simulink model "LAB3"  (R2023a)
settings: Solver=VariableStepAuto  StartTime=0.0  StopTime=10.0  MaxStep=0.001  RelTol=1e-3
values from neighbouring files (symbols this model uses):
  K = 1.5    [LAB3.m]
  T = 0.5    [LAB3.m]
  Wn = 8    [LAB3.m]
  Zeta = 1    [LAB3.m]
settings Model: Creator=alaam  LastModifiedBy=alaam

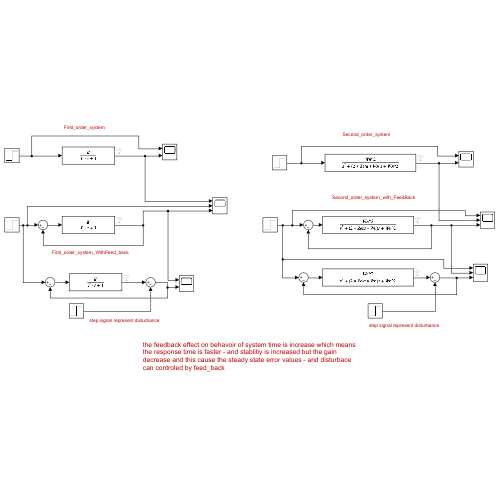
[thumbnail: Simulink's stored preview of the top-level diagram]
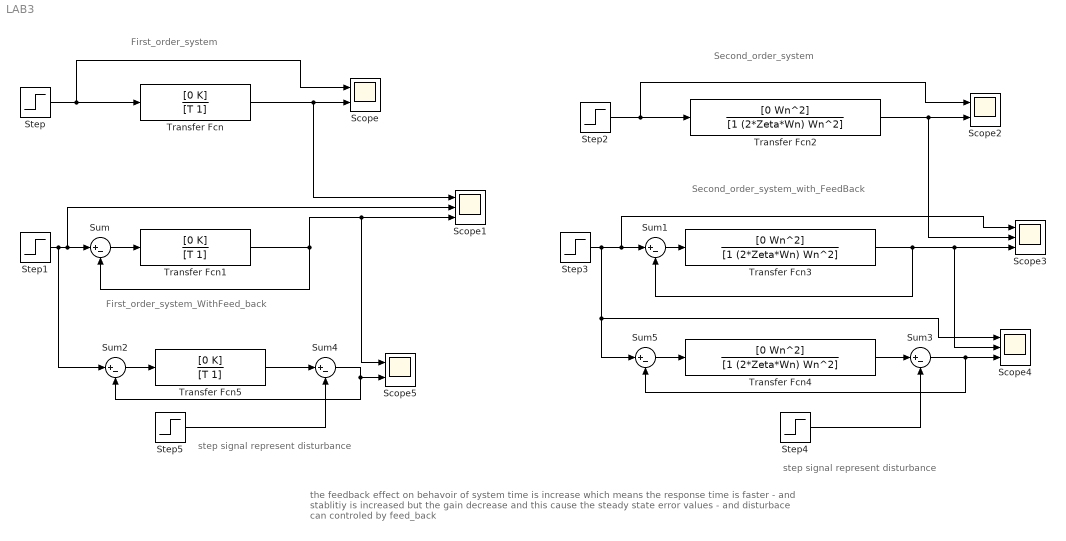
== system LAB3 ==
  note: the feedback effect on behavoir of system time is increase which means the response time is faster - and stablitiy is increased but the gain decrease and this cause the steady state error values - and disturbace can controled by feed_back
  note: step signal represent disturbance
  note: First_order_system
  note: First_order_system_WithFeed_back
  note: Second_order_system
  note: Second_order_system_with_FeedBack
  note: step signal represent disturbance
  Scope : Scope  NumInputPorts=2
  Scope1 : Scope  NumInputPorts=3
  Scope2 : Scope  NumInputPorts=2
  Scope3 : Scope  NumInputPorts=3
  Scope4 : Scope  NumInputPorts=3
  Scope5 : Scope  NumInputPorts=2
  Step{,1..3} (4 alike) : Step  SampleTime=0
  Step4 : Step  Time=5  After=0.3  SampleTime=0
  Step5 : Step  Time=3  After=0.8  SampleTime=0
  Sum{,1..5} (6 alike) : Sum  Inputs=|+-
  Transfer Fcn : TransferFcn  Numerator=[0 K]  Denominator=[T 1]
  Transfer Fcn1 : TransferFcn  Numerator=[0 K]  Denominator=[T 1]
  Transfer Fcn2 : TransferFcn  Numerator=[0 Wn^2]  Denominator=[1 (2*Zeta*Wn) Wn^2]
  Transfer Fcn3 : TransferFcn  Numerator=[0 Wn^2]  Denominator=[1 (2*Zeta*Wn) Wn^2]
  Transfer Fcn4 : TransferFcn  Numerator=[0 Wn^2]  Denominator=[1 (2*Zeta*Wn) Wn^2]
  Transfer Fcn5 : TransferFcn  Numerator=[0 K]  Denominator=[T 1]
  wires:
  Transfer Fcn/1 -> Scope1/1, Scope/2
  Step/1 -> Scope/1, Transfer Fcn/1
  Transfer Fcn1/1 -> Sum/2, Scope1/3, Scope5/1
  Sum/1 -> Transfer Fcn1/1
  Step2/1 -> Scope2/1, Transfer Fcn2/1
  Transfer Fcn2/1 -> Scope3/2, Scope2/2
  Transfer Fcn3/1 -> Sum1/2, Scope4/2, Scope3/3
  Sum1/1 -> Transfer Fcn3/1
  Step3/1 -> Scope4/1, Sum5/1, Scope3/1, Sum1/1
  Transfer Fcn4/1 -> Sum3/1
  Step4/1 -> Sum3/2
  Sum3/1 -> Scope4/3, Sum5/2
  Sum2/1 -> Transfer Fcn5/1
  Transfer Fcn5/1 -> Sum4/1
  Step1/1 -> Sum2/1, Sum/1, Scope1/2
  Step5/1 -> Sum4/2
  Sum4/1 -> Sum2/2, Scope5/2
  Sum5/1 -> Transfer Fcn4/1
